simulink model "MATLAB_TEST"  (R2019b)
settings: Solver=FixedStepDiscrete  StartTime=0  StopTime=50  FixedStep=0.0025  RelTol=1e-3
undefined symbols (not defined in the file): BCM_COM_PROC_P20, BCM_COM_PROC_P20_SFW_R2018b, BCM_COM_PROC_P2_5, BCM_COM_PROC_P2_5_SFW_R2018b, BCM_COM_PROC_P5, BCM_COM_PROC_P5_SFW_R2018b, BCMA_ACCU_PT_Conf_Flt, BCMA_ACCU_PT_Unconf_Flt, BCMA_Antiskid_Off_Sanction, BCMA_Avionics_Conf_Flt, BCMA_BCM_CCDL_Conf_Flt, BCMA_BCM_CCDL_Unconf_Flt, BCMA_BCM_DBCU_INHIBITION_Conf_Flt, BCMA_BCM_DBCU_INHIBITION_Unconf_Flt, BCMA_BCP_ALT_Disp_Sw_Conf_Flt, BCMA_BCP_ALT_Disp_Sw_Unconf_Flt, BCMA_BCP_ALT_SW_ON_CMD_Conf_Flt, BCMA_BCP_ALT_SW_ON_CMD_Unconf_Flt, BCMA_BCP_PARK_OFF_SW_CMD_Conf_Flt, BCMA_BCP_PARK_OFF_SW_CMD_Unconf_Flt, BCMA_CF_BSELV_JCL, BCMA_CF_BSELV_JOP, BCMA_CF_BSELV_OC, BCMA_CF_BSELV_SC, BCMA_CF_LH_SV_JCL, BCMA_CF_LH_SV_JOP, BCMA_CF_LH_SV_OC, BCMA_CF_LH_SV_SC, BCMA_CF_PARK_BRK, BCMA_CF_RESIDUAL_PRESS, BCMA_CF_RH_SV_JCL, BCMA_CF_RH_SV_JOP, BCMA_CF_RH_SV_OC, BCMA_CF_RH_SV_SC, BCMA_CF_SELV_JCL, BCMA_CF_SELV_JOP, BCMA_CF_SELV_OC, BCMA_CF_SELV_SC, BCMA_CF_SV_DRIFT, BCMA_DBCU_ALT_MODE_Conf_Flt, BCMA_DBCU_ALT_MODE_Unconf_Flt, BCMA_DBCU_BRK_ORDER_FAIL_Conf_Flt, BCMA_DBCU_BRK_ORDER_FAIL_Unconf_Flt, BCMA_DBCU_Conf_Flt, BCMA_DBCU_DISPATCH_SW_ON_Conf_Flt, BCMA_DBCU_DISPATCH_SW_ON_Unconf_Flt, BCMA_DBCU_FAILED_Conf_Flt, BCMA_DBCU_FAILED_Unconf_Flt, BCMA_DFCS1_Capsule_Validity, BCMA_DFCS1_Label202_Corrupted, BCMA_DFCS1_Label202_Not_Refreshed, BCMA_DFCS1_Label204_Corrupted, BCMA_DFCS1_Label204_Not_Refreshed, BCMA_DFCS1_Label205_Corrupted, BCMA_DFCS1_Label205_Not_Refreshed, BCMA_DFCS1_Label206_Corrupted, BCMA_DFCS1_Label206_Not_Refreshed, BCMA_DFCS1_Label207_Corrupted, BCMA_DFCS1_Label207_Not_Refreshed, BCMA_DFCS3_Capsule_Validity ... (+762)
libraries: simulink x73, lib_MBD_Control x5
(part 6 of 16)

== system MATLAB_TEST/AVIONICS/Brake_Control_Module_Side_A/BCSA Controller CP/BCM_COM_PROC_P2_5 ==
  V_BCM_COM_Tacho_Acq_W12 : Inport
  V_BCM_COM_Tacho_Unconf_Flt_W12 : Inport  Port=2
  V_BCM_COM_Tacho_Conf_Flt_W12 : Inport  Port=3
  V_BCM_COM_Tacho_Acq_W34 : Inport  Port=4
  V_BCM_COM_Tacho_Unconf_Flt_W34 : Inport  Port=5
  V_BCM_COM_Tacho_Conf_Flt_W34 : Inport  Port=6
  V_BCM_COM_Whl_LP_AS_Curr_Order_W12 : Inport  Port=7
  V_BCM_COM_Press_Cmd_Rate_Lim : Inport  Port=8
  V_BCM_COM_Whl_LP_AS_Curr_Order_W34 : Inport  Port=9
  V_BCM_COM_Global_Reference_Spd : Inport  Port=10
  V_BCM_COM_Wheels_Global_Spun_Up_Ste : Inport  Port=11
  BCM_Tuning : Inport  Port=12
  Enable : EnablePort  StatesWhenEnabling=reset
      settings: AttributesFormatString=StatesWhenEnabling %<StatesWhenEnabling>
  BCM_COM_PROC_P2_5 : Subsystem  Priority=1  AncestorBlock=BCM_COM_PROC_P2_5_SFW_R2018b/BCM_COM_PROC_P2_5  TreatAsAtomicUnit=on  SystemSampleTime=0.0025
  V_BCM_COM_Wheel_Speed_Cons_W12 : Outport
  V_BCM_COM_Wheel_Speed_W12 : Outport  Port=2
  V_BCM_COM_Wheel_Speed_Val_W12 : Outport  Port=3
  V_BCM_COM_Wheel_Speed_Cons_W34 : Outport  Port=4
  V_BCM_COM_Wheel_Speed_W34 : Outport  Port=5
  V_BCM_COM_Wheel_Speed_Val_W34 : Outport  Port=6
  V_BCM_COM_Whl_Filt_Spd_For_AS_W12 : Outport  Port=7
  V_BCM_COM_Wheel_Filtered_Speed_W12 : Outport  Port=8
  V_BCM_COM_Min_Last_8_Whl_Spd_W12 : Outport  Port=9
  V_BCM_COM_Max_Last_8_Whl_Spd_W12 : Outport  Port=10
  V_BCM_COM_Whl_Filt_Spd_For_AS_W34 : Outport  Port=11
  V_BCM_COM_Wheel_Filtered_Speed_W34 : Outport  Port=12
  V_BCM_COM_Min_Last_8_Whl_Spd_W34 : Outport  Port=13
  V_BCM_COM_Max_Last_8_Whl_Spd_W34 : Outport  Port=14
  V_BCM_COM_DCL_Acc : Outport  Port=15
  V_BCM_COM_CT_BCS_WS_First_Filter : Outport  Port=16
  wires:
  V_BCM_COM_Tacho_Acq_W12/1 -> BCM_COM_PROC_P2_5/1(V_BCM_COM_Tacho_Acq_W12)
  V_BCM_COM_Tacho_Unconf_Flt_W12/1 -> BCM_COM_PROC_P2_5/2(V_BCM_COM_Tacho_Unconf_Flt_W12)
  V_BCM_COM_Tacho_Conf_Flt_W12/1 -> BCM_COM_PROC_P2_5/3(V_BCM_COM_Tacho_Conf_Flt_W12)
  V_BCM_COM_Tacho_Acq_W34/1 -> BCM_COM_PROC_P2_5/4(V_BCM_COM_Tacho_Acq_W34)
  V_BCM_COM_Tacho_Unconf_Flt_W34/1 -> BCM_COM_PROC_P2_5/5(V_BCM_COM_Tacho_Unconf_Flt_W34)
  V_BCM_COM_Tacho_Conf_Flt_W34/1 -> BCM_COM_PROC_P2_5/6(V_BCM_COM_Tacho_Conf_Flt_W34)
  BCM_COM_PROC_P2_5/1(V_BCM_COM_Wheel_Speed_Cons_W12) -> V_BCM_COM_Wheel_Speed_Cons_W12/1
  BCM_COM_PROC_P2_5/2(V_BCM_COM_Wheel_Speed_W12) -> V_BCM_COM_Wheel_Speed_W12/1
  BCM_COM_PROC_P2_5/3(V_BCM_COM_Wheel_Speed_Val_W12) -> V_BCM_COM_Wheel_Speed_Val_W12/1
  BCM_COM_PROC_P2_5/4(V_BCM_COM_Wheel_Speed_Cons_W34) -> V_BCM_COM_Wheel_Speed_Cons_W34/1
  BCM_COM_PROC_P2_5/5(V_BCM_COM_Wheel_Speed_W34) -> V_BCM_COM_Wheel_Speed_W34/1
  BCM_COM_PROC_P2_5/6(V_BCM_COM_Wheel_Speed_Val_W34) -> V_BCM_COM_Wheel_Speed_Val_W34/1
  BCM_COM_PROC_P2_5/7(V_BCM_COM_Whl_Filt_Spd_For_AS_W12) -> V_BCM_COM_Whl_Filt_Spd_For_AS_W12/1
  BCM_COM_PROC_P2_5/8(V_BCM_COM_Wheel_Filtered_Speed_W12) -> V_BCM_COM_Wheel_Filtered_Speed_W12/1
  BCM_COM_PROC_P2_5/9(V_BCM_COM_Min_Last_8_Whl_Spd_W12) -> V_BCM_COM_Min_Last_8_Whl_Spd_W12/1
  BCM_COM_PROC_P2_5/10(V_BCM_COM_Max_Last_8_Whl_Spd_W12) -> V_BCM_COM_Max_Last_8_Whl_Spd_W12/1
  BCM_COM_PROC_P2_5/11(V_BCM_COM_Whl_Filt_Spd_For_AS_W34) -> V_BCM_COM_Whl_Filt_Spd_For_AS_W34/1
  BCM_COM_PROC_P2_5/12(V_BCM_COM_Wheel_Filtered_Speed_W34) -> V_BCM_COM_Wheel_Filtered_Speed_W34/1
  BCM_COM_PROC_P2_5/13(V_BCM_COM_Min_Last_8_Whl_Spd_W34) -> V_BCM_COM_Min_Last_8_Whl_Spd_W34/1
  BCM_COM_PROC_P2_5/14(V_BCM_COM_Max_Last_8_Whl_Spd_W34) -> V_BCM_COM_Max_Last_8_Whl_Spd_W34/1
  V_BCM_COM_Whl_LP_AS_Curr_Order_W34/1 -> BCM_COM_PROC_P2_5/9(V_BCM_COM_Whl_LP_AS_Curr_Order_W34)
  V_BCM_COM_Press_Cmd_Rate_Lim/1 -> BCM_COM_PROC_P2_5/8(V_BCM_COM_Press_Cmd_Rate_Lim)
  V_BCM_COM_Whl_LP_AS_Curr_Order_W12/1 -> BCM_COM_PROC_P2_5/7(V_BCM_COM_Whl_LP_AS_Curr_Order_W12)
  BCM_Tuning/1 -> BCM_COM_PROC_P2_5/12(BCM_Tuning)
  V_BCM_COM_Wheels_Global_Spun_Up_Ste/1 -> BCM_COM_PROC_P2_5/11(V_BCM_COM_Wheels_Global_Spun_Up_Ste)
  V_BCM_COM_Global_Reference_Spd/1 -> BCM_COM_PROC_P2_5/10(V_BCM_COM_Global_Reference_Spd)
  BCM_COM_PROC_P2_5/15(V_BCM_COM_DCL_Acc) -> V_BCM_COM_DCL_Acc/1
  BCM_COM_PROC_P2_5/16(V_BCM_COM_CT_BCS_WS_First_Filter) -> V_BCM_COM_CT_BCS_WS_First_Filter/1

== system MATLAB_TEST/AVIONICS/Brake_Control_Module_Side_A/BCSA Controller CP/BCM_COM_PROC_P5 ==
  V_BCM_COM_LH_SV_PT_Acq : Inport
  V_BCM_COM_RH_SV_PT_Acq : Inport  Port=2
  V_BCM_COM_LH_SV_PT_Unconf_Flt : Inport  Port=3
  V_BCM_COM_RH_SV_PT_Unconf_Flt : Inport  Port=4
  V_BCM_COM_LH_SV_PT_Conf_Flt : Inport  Port=5
  V_BCM_COM_RH_SV_PT_Conf_Flt : Inport  Port=6
  V_BCM_COM_BCM_Config : Inport  Port=7
  V_BCM_COM_Brkg_On_Wheels : Inport  Port=8
  V_BCM_COM_Press_Cmd_Rate_Lim : Inport  Port=9
  V_BCM_COM_SELV_High_Side_Cmd_Order : Inport  Port=10
  V_BCM_COM_PBSELV_State_Cons : Inport  Port=11
  V_BCM_COM_Braking_State : Inport  Port=12
  V_BCM_COM_LH_Press_Reg_FT_Act_Cond : Inport  Port=13
  V_BCM_COM_RH_Press_Reg_FT_Act_Cond : Inport  Port=14
  V_BCM_COM_Braking_Mode : Inport  Port=15
  V_BCM_COM_Whl_Filt_Spd_For_AS_W12 : Inport  Port=16
  V_BCM_COM_Whl_Filt_Spd_For_AS_W34 : Inport  Port=17
  V_BCM_COM_Tacho_Conf_Flt_W12 : Inport  Port=18
  V_BCM_COM_Tacho_Conf_Flt_W34 : Inport  Port=19
  V_BCM_COM_AC_State : Inport  Port=20
  V_BCM_COM_AC_Flight_Phase : Inport  Port=21
  V_BCM_COM_UF_LOCKED_WHEEL_W12 : Inport  Port=22
  V_BCM_COM_UF_LOCKED_WHEEL_W34 : Inport  Port=23
  V_BCM_COM_Wheel_Control_Speed_W12 : Inport  Port=24
  V_BCM_COM_Wheel_Control_Speed_W34 : Inport  Port=25
  V_BCM_COM_Whl_AS_Adp_Gain_W12 : Inport  Port=26
  V_BCM_COM_Whl_AS_Adp_Gain_W34 : Inport  Port=27
  V_BCM_COM_Decel_Ctrl_Loop_Act_Cond : Inport  Port=28
  V_BCM_COM_Wheels_Global_Spun_Up_Ste : Inport  Port=29
  V_BCM_COM_Global_Reference_Spd : Inport  Port=30
  V_BCM_COM_LH_Press_Law_Brkg_Press_Cmd : Inport  Port=31
  V_BCM_COM_RH_Press_Law_Brkg_Press_Cmd : Inport  Port=32
  V_BCM_COM_Target_DCL : Inport  Port=33
  V_BCM_COM_DCL_Acc : Inport  Port=34
  BCM_Tuning : Inport  Port=35
  Enable : EnablePort  StatesWhenEnabling=reset
      settings: AttributesFormatString=StatesWhenEnabling %<StatesWhenEnabling>
  BCM_COM_PROC_P5 : Subsystem  Priority=2  AncestorBlock=BCM_COM_PROC_P5_SFW_R2018b/BCM_COM_PROC_P5  TreatAsAtomicUnit=on  SystemSampleTime=0.005
  V_BCM_COM_SV_PT_Cons : Outport
  V_BCM_COM_SV_PT_Cons_Val : Outport  Port=2
  V_BCM_COM_SV_Current : Outport  Port=3
  V_BCM_COM_SV_Curr_AS_Protect : Outport  Port=4
  V_BCM_COM_SV_Current_Order : Outport  Port=5
  V_BCM_COM_SV_PT_Filt : Outport  Port=6
  V_BCM_COM_Corr_Press_Cmd : Outport  Port=7
  V_BCM_COM_SV_Drift : Outport  Port=8
  V_BCM_COM_PCL_State : Outport  Port=9
  V_BCM_COM_Whl_AS_Activity : Outport  Port=10
  V_BCM_COM_Press_Reg_Act_Cond : Outport  Port=11
  V_BCM_COM_Whl_LP_AS_Curr_Order_W12 : Outport  Port=12  VectorParamsAs1DForOutWhenUnconnected=off
  V_BCM_COM_Whl_LP_AS_Curr_Order_W34 : Outport  Port=13  VectorParamsAs1DForOutWhenUnconnected=off
  V_BCM_COM_Whl_AS_Inhib_Cond_W12 : Outport  Port=14  VectorParamsAs1DForOutWhenUnconnected=off
  V_BCM_COM_Whl_AS_Inhib_Cond_W34 : Outport  Port=15  VectorParamsAs1DForOutWhenUnconnected=off
  V_BCM_COM_Whl_LP_AS_Curr_Order : Outport  Port=16  VectorParamsAs1DForOutWhenUnconnected=off
  V_BCM_COM_Wheel_Speed_Error_W12 : Outport  Port=17  VectorParamsAs1DForOutWhenUnconnected=off
  V_BCM_COM_Wheel_Speed_Error_W34 : Outport  Port=18  VectorParamsAs1DForOutWhenUnconnected=off
  V_BCM_COM_Whl_AS_Curr_Order : Outport  Port=19  VectorParamsAs1DForOutWhenUnconnected=off
  V_BCM_COM_LH_Decel_Law_Brkg_Press_Cmd : Outport  Port=20
  V_BCM_COM_RH_Decel_Law_Brkg_Press_Cmd : Outport  Port=21
  wires:
  V_BCM_COM_LH_SV_PT_Acq/1 -> BCM_COM_PROC_P5/1(V_BCM_COM_LH_SV_PT_Acq)
  V_BCM_COM_RH_SV_PT_Acq/1 -> BCM_COM_PROC_P5/2(V_BCM_COM_RH_SV_PT_Acq)
  V_BCM_COM_LH_SV_PT_Unconf_Flt/1 -> BCM_COM_PROC_P5/3(V_BCM_COM_LH_SV_PT_Unconf_Flt)
  V_BCM_COM_RH_SV_PT_Unconf_Flt/1 -> BCM_COM_PROC_P5/4(V_BCM_COM_RH_SV_PT_Unconf_Flt)
  V_BCM_COM_LH_SV_PT_Conf_Flt/1 -> BCM_COM_PROC_P5/5(V_BCM_COM_LH_SV_PT_Conf_Flt)
  V_BCM_COM_RH_SV_PT_Conf_Flt/1 -> BCM_COM_PROC_P5/6(V_BCM_COM_RH_SV_PT_Conf_Flt)
  V_BCM_COM_BCM_Config/1 -> BCM_COM_PROC_P5/7(V_BCM_COM_BCM_Config)
  V_BCM_COM_Brkg_On_Wheels/1 -> BCM_COM_PROC_P5/8(V_BCM_COM_Brkg_On_Wheels)
  V_BCM_COM_Press_Cmd_Rate_Lim/1 -> BCM_COM_PROC_P5/9(V_BCM_COM_Press_Cmd_Rate_Lim)
  V_BCM_COM_SELV_High_Side_Cmd_Order/1 -> BCM_COM_PROC_P5/10(V_BCM_COM_SELV_High_Side_Cmd_Order)
  V_BCM_COM_PBSELV_State_Cons/1 -> BCM_COM_PROC_P5/11(V_BCM_COM_PBSELV_State_Cons)
  V_BCM_COM_Braking_State/1 -> BCM_COM_PROC_P5/12(V_BCM_COM_Braking_State)
  V_BCM_COM_LH_Press_Reg_FT_Act_Cond/1 -> BCM_COM_PROC_P5/13(V_BCM_COM_LH_Press_Reg_FT_Act_Cond)
  V_BCM_COM_RH_Press_Reg_FT_Act_Cond/1 -> BCM_COM_PROC_P5/14(V_BCM_COM_RH_Press_Reg_FT_Act_Cond)
  V_BCM_COM_Braking_Mode/1 -> BCM_COM_PROC_P5/15(V_BCM_COM_Braking_Mode)
  V_BCM_COM_Whl_Filt_Spd_For_AS_W12/1 -> BCM_COM_PROC_P5/16(V_BCM_COM_Whl_Filt_Spd_For_AS_W12)
  V_BCM_COM_Whl_Filt_Spd_For_AS_W34/1 -> BCM_COM_PROC_P5/17(V_BCM_COM_Whl_Filt_Spd_For_AS_W34)
  V_BCM_COM_Tacho_Conf_Flt_W12/1 -> BCM_COM_PROC_P5/18(V_BCM_COM_Tacho_Conf_Flt_W12)
  V_BCM_COM_Tacho_Conf_Flt_W34/1 -> BCM_COM_PROC_P5/19(V_BCM_COM_Tacho_Conf_Flt_W34)
  V_BCM_COM_AC_State/1 -> BCM_COM_PROC_P5/20(V_BCM_COM_AC_State)
  V_BCM_COM_AC_Flight_Phase/1 -> BCM_COM_PROC_P5/21(V_BCM_COM_AC_Flight_Phase)
  V_BCM_COM_UF_LOCKED_WHEEL_W12/1 -> BCM_COM_PROC_P5/22(V_BCM_COM_UF_LOCKED_WHEEL_W12)
  V_BCM_COM_UF_LOCKED_WHEEL_W34/1 -> BCM_COM_PROC_P5/23(V_BCM_COM_UF_LOCKED_WHEEL_W34)
  V_BCM_COM_Wheel_Control_Speed_W12/1 -> BCM_COM_PROC_P5/24(V_BCM_COM_Wheel_Control_Speed_W12)
  V_BCM_COM_Wheel_Control_Speed_W34/1 -> BCM_COM_PROC_P5/25(V_BCM_COM_Wheel_Control_Speed_W34)
  V_BCM_COM_Whl_AS_Adp_Gain_W12/1 -> BCM_COM_PROC_P5/26(V_BCM_COM_Whl_AS_Adp_Gain_W12)
  V_BCM_COM_Whl_AS_Adp_Gain_W34/1 -> BCM_COM_PROC_P5/27(V_BCM_COM_Whl_AS_Adp_Gain_W34)
  V_BCM_COM_Decel_Ctrl_Loop_Act_Cond/1 -> BCM_COM_PROC_P5/28(V_BCM_COM_Decel_Ctrl_Loop_Act_Cond)
  V_BCM_COM_Wheels_Global_Spun_Up_Ste/1 -> BCM_COM_PROC_P5/29(V_BCM_COM_Wheels_Global_Spun_Up_Ste)
  V_BCM_COM_Global_Reference_Spd/1 -> BCM_COM_PROC_P5/30(V_BCM_COM_Global_Reference_Spd)
  V_BCM_COM_LH_Press_Law_Brkg_Press_Cmd/1 -> BCM_COM_PROC_P5/31(V_BCM_COM_LH_Press_Law_Brkg_Press_Cmd)
  V_BCM_COM_RH_Press_Law_Brkg_Press_Cmd/1 -> BCM_COM_PROC_P5/32(V_BCM_COM_RH_Press_Law_Brkg_Press_Cmd)
  V_BCM_COM_Target_DCL/1 -> BCM_COM_PROC_P5/33(V_BCM_COM_Target_DCL)
  V_BCM_COM_DCL_Acc/1 -> BCM_COM_PROC_P5/34(V_BCM_COM_DCL_Acc)
  BCM_Tuning/1 -> BCM_COM_PROC_P5/35(BCM_Tuning)
  BCM_COM_PROC_P5/1(V_BCM_COM_SV_PT_Cons) -> V_BCM_COM_SV_PT_Cons/1
  BCM_COM_PROC_P5/2(V_BCM_COM_SV_PT_Cons_Val) -> V_BCM_COM_SV_PT_Cons_Val/1
  BCM_COM_PROC_P5/3(V_BCM_COM_SV_Current) -> V_BCM_COM_SV_Current/1
  BCM_COM_PROC_P5/4(V_BCM_COM_SV_Curr_AS_Protect) -> V_BCM_COM_SV_Curr_AS_Protect/1
  BCM_COM_PROC_P5/5(V_BCM_COM_SV_Current_Order) -> V_BCM_COM_SV_Current_Order/1
  BCM_COM_PROC_P5/6(V_BCM_COM_SV_PT_Filt) -> V_BCM_COM_SV_PT_Filt/1
  BCM_COM_PROC_P5/7(V_BCM_COM_Corr_Press_Cmd) -> V_BCM_COM_Corr_Press_Cmd/1
  BCM_COM_PROC_P5/8(V_BCM_COM_PCL_State) -> V_BCM_COM_PCL_State/1
  BCM_COM_PROC_P5/9(V_BCM_COM_Whl_AS_Activity) -> V_BCM_COM_Whl_AS_Activity/1
  BCM_COM_PROC_P5/10(V_BCM_COM_Press_Reg_Act_Cond) -> V_BCM_COM_Press_Reg_Act_Cond/1
  BCM_COM_PROC_P5/11(V_BCM_COM_Whl_LP_AS_Curr_Order_W12) -> V_BCM_COM_Whl_LP_AS_Curr_Order_W12/1
  BCM_COM_PROC_P5/12(V_BCM_COM_Whl_LP_AS_Curr_Order_W34) -> V_BCM_COM_Whl_LP_AS_Curr_Order_W34/1
  BCM_COM_PROC_P5/13(V_BCM_COM_Whl_AS_Inhib_Cond_W12) -> V_BCM_COM_Whl_AS_Inhib_Cond_W12/1
  BCM_COM_PROC_P5/14(V_BCM_COM_Whl_AS_Inhib_Cond_W34) -> V_BCM_COM_Whl_AS_Inhib_Cond_W34/1
  BCM_COM_PROC_P5/15(V_BCM_COM_Whl_LP_AS_Curr_Order) -> V_BCM_COM_Whl_LP_AS_Curr_Order/1
  BCM_COM_PROC_P5/16(V_BCM_COM_Wheel_Speed_Error_W12) -> V_BCM_COM_Wheel_Speed_Error_W12/1
  BCM_COM_PROC_P5/17(V_BCM_COM_Wheel_Speed_Error_W34) -> V_BCM_COM_Wheel_Speed_Error_W34/1
  BCM_COM_PROC_P5/18(V_BCM_COM_Whl_AS_Curr_Order) -> V_BCM_COM_Whl_AS_Curr_Order/1
  BCM_COM_PROC_P5/19(V_BCM_COM_SV_Drift) -> V_BCM_COM_SV_Drift/1
  BCM_COM_PROC_P5/20(V_BCM_COM_LH_Decel_Law_Brkg_Press_Cmd) -> V_BCM_COM_LH_Decel_Law_Brkg_Press_Cmd/1
  BCM_COM_PROC_P5/21(V_BCM_COM_RH_Decel_Law_Brkg_Press_Cmd) -> V_BCM_COM_RH_Decel_Law_Brkg_Press_Cmd/1

== system MATLAB_TEST/AVIONICS/Brake_Control_Module_Side_A/BCSA Controller CP/BUS_A429_BCMA_DFCS13_TX ==
  note: Emission rate 80 Hz TBC
  BCMCP_LH_Braking_Cmd_Feedback : Inport
  BCMCP_RH_Braking_Cmd_Feedback : Inport  Port=2
  BCMCP_LHO_Wheel_Speed : Inport  Port=3
  BCMCP_LHI_Wheel_Speed : Inport  Port=4
  BCMCP_RHI_Wheel_Speed : Inport  Port=5
  BCMCP_RHO_Wheel_Speed : Inport  Port=6
  BCMCP_DFCS_Caps_1_Fail : Inport  Port=7  OutDataTypeStr=boolean
  BCMCP_DFCS_Caps_2_Fail : Inport  Port=8  OutDataTypeStr=boolean
  BCMCP_BCM_Failed : Inport  Port=9
  BCMCP_BCM_Passivated : Inport  Port=10
  BCMCP_Preland_Test : Inport  Port=11
  BCMCP_Retract_Test : Inport  Port=12
  BCMCP_Braking_Request : Inport  Port=13
  BCMCP_Antiskid_Active : Inport  Port=14
  BCMCP_LH_Brake_Pressure : Inport  Port=15
  BCMCP_RH_Brake_Pressure : Inport  Port=16
  BCMSP_LHO_Wheel_Speed : Inport  Port=17
  BCMSP_LHI_Wheel_Speed : Inport  Port=18
  BCMSP_RHI_Wheel_Speed : Inport  Port=19
  BCMSP_RHO_Wheel_Speed : Inport  Port=20
  BCMSP_LH_Brake_Pressure : Inport  Port=21
  BCMSP_RH_Brake_Pressure : Inport  Port=22
  BCMSP_LH_Braking_Cmd_Feedback : Inport  Port=23
  BCMSP_RH_Braking_Cmd_Feedback : Inport  Port=24
  BCMSP_DFCS_Caps_1_Fail : Inport  Port=25  OutDataTypeStr=boolean
  BCMSP_DFCS_Caps_2_Fail : Inport  Port=26  OutDataTypeStr=boolean
  BCMSP_BCM_Failed : Inport  Port=27
  BCMSP_BCM_Passivated : Inport  Port=28
  LABEL_100_SSM : Inport  Port=29
  LABEL_101_SSM : Inport  Port=30
  LABEL_102_SSM : Inport  Port=31
  LABEL_103_SSM : Inport  Port=32
  LABEL_104_SSM : Inport  Port=33
  LABEL_105_SSM : Inport  Port=34
  LABEL_106_SSM : Inport  Port=35
  LABEL_107_SSM : Inport  Port=36
  LABEL_121_SSM : Inport  Port=37
  LABEL_122_SSM : Inport  Port=38
  LABEL_123_SSM : Inport  Port=39
  LABEL_124_SSM : Inport  Port=40
  LABEL_125_SSM : Inport  Port=41
  LABEL_126_SSM : Inport  Port=42
  LABEL_127_SSM : Inport  Port=43
  LABEL_130_SSM : Inport  Port=44
  LABEL_131_SSM : Inport  Port=45
  LABEL_150_SSM : Inport  Port=46
  LABEL_151_SSM : Inport  Port=47
  Bus Creator : BusCreator  Inputs=50  OutDataTypeStr=Bus: SMLK_BUS_A429_BCMA_DFCS13  NonVirtualBus=on
      settings: InheritFromInputs=off
  LABEL_121_Counter : Constant  Value=0  OutDataTypeStr=uint32
  LABEL_150_CRC_MSW : Constant  Value=0  OutDataTypeStr=uint32
  LABEL_151_CRC_LSW : Constant  Value=0  OutDataTypeStr=uint32
  Rate Transition{2..51} (50 alike) : RateTransition  Deterministic=off  OutPortSampleTime=1/80
      settings: AttributesFormatString=OutPortSampleTime %<OutPortSampleTime>
  BUS_A429_BCMA_DFCS13 : Outport  VectorParamsAs1DForOutWhenUnconnected=off
  wires:
  LABEL_100_SSM/1 -> Rate Transition2/1  "BUS_A429_BCMA_DFCS13_LABEL_100_SSM"
  BCMCP_LH_Braking_Cmd_Feedback/1 -> Rate Transition3/1  "BUS_A429_BCMA_DFCS13_LABEL_100_BCMCP_LH_Braking_Cmd_Feedback"
  BCMCP_RH_Braking_Cmd_Feedback/1 -> Rate Transition4/1  "BUS_A429_BCMA_DFCS13_LABEL_100_BCMCP_RH_Braking_Cmd_Feedback"
  LABEL_101_SSM/1 -> Rate Transition5/1  "BUS_A429_BCMA_DFCS13_LABEL_101_SSM"
  LABEL_102_SSM/1 -> Rate Transition7/1  "BUS_A429_BCMA_DFCS13_LABEL_102_SSM"
  LABEL_103_SSM/1 -> Rate Transition9/1  "BUS_A429_BCMA_DFCS13_LABEL_103_SSM"
  LABEL_104_SSM/1 -> Rate Transition11/1  "BUS_A429_BCMA_DFCS13_LABEL_104_SSM"
  LABEL_105_SSM/1 -> Rate Transition13/1  "BUS_A429_BCMA_DFCS13_LABEL_105_SSM"
  BCMCP_LHI_Wheel_Speed/1 -> Rate Transition6/1  "BUS_A429_BCMA_DFCS13_LABEL_101_BCMCP_LHI_Wheel_Speed"
  BCMCP_RHI_Wheel_Speed/1 -> Rate Transition8/1  "BUS_A429_BCMA_DFCS13_LABEL_102_BCMCP_RHI_Wheel_Speed"
  BCMCP_LHO_Wheel_Speed/1 -> Rate Transition10/1  "BUS_A429_BCMA_DFCS13_LABEL_103_BCMCP_LHO_Wheel_Speed"
  BCMCP_RHO_Wheel_Speed/1 -> Rate Transition12/1  "BUS_A429_BCMA_DFCS13_LABEL_104_BCMCP_RHO_Wheel_Speed"
  BCMCP_DFCS_Caps_1_Fail/1 -> Rate Transition14/1  "BUS_A429_BCMA_DFCS13_LABEL_105_DATA_BIT_11_BCMCP_DFCS_Caps_1_Fail"
  BCMCP_DFCS_Caps_2_Fail/1 -> Rate Transition15/1  "BUS_A429_BCMA_DFCS13_LABEL_105_DATA_BIT_12_BCMCP_DFCS_Caps_2_Fail"
  BCMCP_BCM_Failed/1 -> Rate Transition16/1  "BUS_A429_BCMA_DFCS13_LABEL_105_DATA_BIT_13_BCMCP_BCM_Failed"
  BCMCP_BCM_Passivated/1 -> Rate Transition17/1  "BUS_A429_BCMA_DFCS13_LABEL_105_DATA_BIT_14_BCMCP_BCM_Passivated"
  BCMCP_Preland_Test/1 -> Rate Transition18/1  "BUS_A429_BCMA_DFCS13_LABEL_105_DATA_BIT_15_BCMCP_Preland_Test"
  BCMCP_Retract_Test/1 -> Rate Transition19/1  "BUS_A429_BCMA_DFCS13_LABEL_105_DATA_BIT_16_BCMCP_Retract_Test"
  BCMCP_Braking_Request/1 -> Rate Transition20/1  "BUS_A429_BCMA_DFCS13_LABEL_105_DATA_BIT_17_BCMCP_Braking_Request"
  BCMCP_Antiskid_Active/1 -> Rate Transition21/1  "BUS_A429_BCMA_DFCS13_LABEL_105_DATA_BIT_18_BCMCP_Antiskid_Active"
  LABEL_106_SSM/1 -> Rate Transition22/1  "BUS_A429_BCMA_DFCS13_LABEL_106_SSM"
  LABEL_107_SSM/1 -> Rate Transition24/1  "BUS_A429_BCMA_DFCS13_LABEL_107_SSM"
  LABEL_121_SSM/1 -> Rate Transition26/1  "BUS_A429_BCMA_DFCS13_LABEL_121_SSM"
  LABEL_123_SSM/1 -> Rate Transition31/1  "BUS_A429_BCMA_DFCS13_LABEL_123_SSM"
  BCMCP_LH_Brake_Pressure/1 -> Rate Transition23/1  "BUS_A429_BCMA_DFCS13_LABEL_106_BCMCP_LH_Brake_Pressure"
  BCMCP_RH_Brake_Pressure/1 -> Rate Transition25/1  "BUS_A429_BCMA_DFCS13_LABEL_107_BCMCP_RH_Brake_Pressure"
  LABEL_122_SSM/1 -> Rate Transition28/1  "BUS_A429_BCMA_DFCS13_LABEL_122_SSM"
  LABEL_121_Counter/1 -> Rate Transition27/1  "BUS_A429_BCMA_DFCS13_LABEL_121_Counter"
  BCMSP_LH_Braking_Cmd_Feedback/1 -> Rate Transition29/1  "BUS_A429_BCMA_DFCS13_LABEL_122_BCMSP_LH_Braking_Cmd_Feedback"
  BCMSP_RH_Braking_Cmd_Feedback/1 -> Rate Transition30/1  "BUS_A429_BCMA_DFCS13_LABEL_122_BCMSP_RH_Braking_Cmd_Feedback"
  BCMSP_LHI_Wheel_Speed/1 -> Rate Transition32/1  "BUS_A429_BCMA_DFCS13_LABEL_123_BCMSP_LHI_Wheel_Speed"
  LABEL_124_SSM/1 -> Rate Transition33/1  "BUS_A429_BCMA_DFCS13_LABEL_124_SSM"
  LABEL_125_SSM/1 -> Rate Transition35/1  "BUS_A429_BCMA_DFCS13_LABEL_125_SSM"
  LABEL_126_SSM/1 -> Rate Transition37/1  "BUS_A429_BCMA_DFCS13_LABEL_126_SSM"
  BCMSP_RHI_Wheel_Speed/1 -> Rate Transition34/1  "BUS_A429_BCMA_DFCS13_LABEL_124_BCMSP_RHI_Wheel_Speed"
  BCMSP_LHO_Wheel_Speed/1 -> Rate Transition36/1  "BUS_A429_BCMA_DFCS13_LABEL_125_BCMSP_LHO_Wheel_Speed"
  BCMSP_RHO_Wheel_Speed/1 -> Rate Transition38/1  "BUS_A429_BCMA_DFCS13_LABEL_126_BCMSP_RHO_Wheel_Speed"
  LABEL_127_SSM/1 -> Rate Transition39/1  "BUS_A429_BCMA_DFCS13_LABEL_127_SSM"
  BCMSP_DFCS_Caps_1_Fail/1 -> Rate Transition40/1  "BUS_A429_BCMA_DFCS13_LABEL_127_DATA_BIT_11_BCMSP_DFCS_Caps_1_Fail"
  BCMSP_DFCS_Caps_2_Fail/1 -> Rate Transition41/1  "BUS_A429_BCMA_DFCS13_LABEL_127_DATA_BIT_12_BCMSP_DFCS_Caps_2_Fail"
  BCMSP_BCM_Failed/1 -> Rate Transition42/1  "BUS_A429_BCMA_DFCS13_LABEL_127_DATA_BIT_13_BCMSP_BCM_Failed"
  BCMSP_BCM_Passivated/1 -> Rate Transition43/1  "BUS_A429_BCMA_DFCS13_LABEL_127_DATA_BIT_14_BCMSP_BCM_Passivated"
  LABEL_130_SSM/1 -> Rate Transition44/1  "BUS_A429_BCMA_DFCS13_LABEL_130_SSM"
  LABEL_131_SSM/1 -> Rate Transition46/1  "BUS_A429_BCMA_DFCS13_LABEL_131_SSM"
  BCMSP_LH_Brake_Pressure/1 -> Rate Transition45/1  "BUS_A429_BCMA_DFCS13_LABEL_130_BCMSP_LH_Brake_Pressure"
  BCMSP_RH_Brake_Pressure/1 -> Rate Transition47/1  "BUS_A429_BCMA_DFCS13_LABEL_131_BCMSP_RH_Brake_Pressure"
  LABEL_150_SSM/1 -> Rate Transition48/1  "BUS_A429_BCMA_DFCS13_LABEL_150_SSM"
  LABEL_150_CRC_MSW/1 -> Rate Transition49/1  "BUS_A429_BCMA_DFCS13_LABEL_150_CRC_MSW"
  LABEL_151_SSM/1 -> Rate Transition50/1  "BUS_A429_BCMA_DFCS13_LABEL_151_SSM"
  LABEL_151_CRC_LSW/1 -> Rate Transition51/1  "BUS_A429_BCMA_DFCS13_LABEL_151_CRC_LSW"
  Bus Creator/1 -> BUS_A429_BCMA_DFCS13/1
  Rate Transition2/1 -> Bus Creator/1
  Rate Transition3/1 -> Bus Creator/2
  Rate Transition4/1 -> Bus Creator/3
  Rate Transition5/1 -> Bus Creator/4
  Rate Transition6/1 -> Bus Creator/5
  Rate Transition7/1 -> Bus Creator/6
  Rate Transition8/1 -> Bus Creator/7
  Rate Transition9/1 -> Bus Creator/8
  Rate Transition10/1 -> Bus Creator/9
  Rate Transition11/1 -> Bus Creator/10
  Rate Transition12/1 -> Bus Creator/11
  Rate Transition13/1 -> Bus Creator/12
  Rate Transition14/1 -> Bus Creator/13
  Rate Transition15/1 -> Bus Creator/14
  Rate Transition16/1 -> Bus Creator/15
  Rate Transition17/1 -> Bus Creator/16
  Rate Transition18/1 -> Bus Creator/17
  Rate Transition19/1 -> Bus Creator/18
  Rate Transition20/1 -> Bus Creator/19
  Rate Transition21/1 -> Bus Creator/20
  Rate Transition22/1 -> Bus Creator/21
  Rate Transition23/1 -> Bus Creator/22
  Rate Transition24/1 -> Bus Creator/23
  Rate Transition25/1 -> Bus Creator/24
  Rate Transition26/1 -> Bus Creator/25
  Rate Transition27/1 -> Bus Creator/26
  Rate Transition28/1 -> Bus Creator/27
  Rate Transition29/1 -> Bus Creator/28
  Rate Transition30/1 -> Bus Creator/29
  Rate Transition31/1 -> Bus Creator/30
  Rate Transition32/1 -> Bus Creator/31
  Rate Transition33/1 -> Bus Creator/32
  Rate Transition34/1 -> Bus Creator/33
  Rate Transition35/1 -> Bus Creator/34
  Rate Transition36/1 -> Bus Creator/35
  Rate Transition37/1 -> Bus Creator/36
  Rate Transition38/1 -> Bus Creator/37
  Rate Transition39/1 -> Bus Creator/38
  Rate Transition40/1 -> Bus Creator/39
  Rate Transition41/1 -> Bus Creator/40
  Rate Transition42/1 -> Bus Creator/41
  Rate Transition43/1 -> Bus Creator/42
  Rate Transition44/1 -> Bus Creator/43
  Rate Transition45/1 -> Bus Creator/44
  Rate Transition46/1 -> Bus Creator/45
  Rate Transition47/1 -> Bus Creator/46
  Rate Transition48/1 -> Bus Creator/47
  Rate Transition49/1 -> Bus Creator/48
  Rate Transition50/1 -> Bus Creator/49
  Rate Transition51/1 -> Bus Creator/50
